simulink model "motorVelMap"  (R2016b)
settings: Solver=ode5  StartTime=0.0  StopTime=inf  FixedStep=0.001  RelTol=1e-3  EnableMultiTasking=on
undefined symbols (not defined in the file or in its folder): Humusoft, MF644
libraries: dcpctrl x2, sldrtlib x1, simulink x1
settings Model: SimulationMode=external  ExtModeArchiveMode=auto  ExtModeArchiveFileName=dsaData  ExtModeArchiveDirName=/Users/julianleland/Documents/Git/GitHub/dcpctrl_v2/data/dsaData  ExtModeIncDirWhenArm=on  Creator=julianleland  LastModifiedBy=julianleland
settings DataIOCC: SaveOutput=off  SignalLogging=off  DSMLogging=off  SaveTime=off
settings OptimizationCC: LifeSpan=inf
settings DebuggingCC: SFUnexpectedBacktrackingDiag=warning  SFNoUnconditionalDefaultTransitionDiag=warning  SFExecutionAtInitializationDiag=none
settings HardwareCC: ProdBitPerLong=64  ProdHWDeviceType=Intel->x86-64 (Mac OS X)  TargetBitPerLong=64  TargetBitPerPointer=64  TargetIntDivRoundTo=Zero  TargetEndianess=LittleEndian  TargetWordSize=64  TargetHWDeviceType=Intel->x86-64
settings RTWCC: SystemTargetFile=sldrt.tlc  TemplateMakefile=sldrt.tmf  Description=Simulink Desktop Real-Time  RTWCompilerOptimization=on
settings CodeAppCC: MaxIdLength=95
settings SimulinkDesktopRealTimeCC: TargetPreCompLibLocation=/Applications/MATLAB_R2016b.app/toolbox/sldrt/lib/maci64  TargetLangStandard=C89/C90 (ANSI)  SupportVariableSizeSignals=off
settings ConfigComp: CovMetricSettings=dw  CovHtmlReporting=on  CovSaveCumulativeToWorkspaceVar=on  CovSaveSingleToWorkspaceVar=on  CovExternalEMLEnable=off

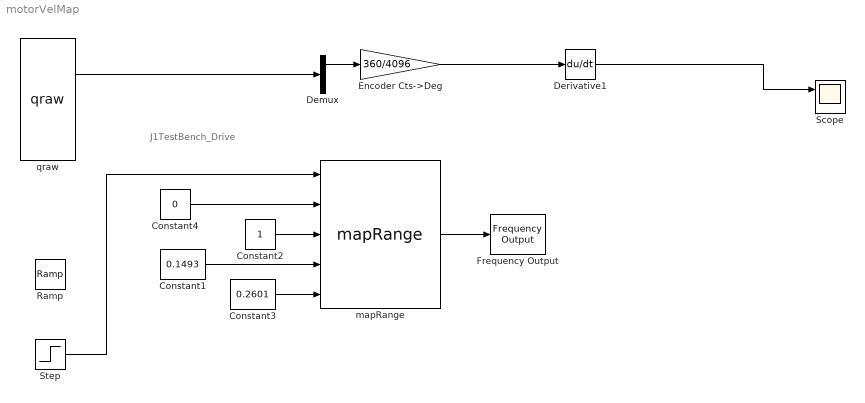
== system motorVelMap ==
  note: J1TestBench_Drive
  Constant1 : Constant  Value=0.1493
  Constant2 : Constant
  Constant3 : Constant  Value=0.2601
  Constant4 : Constant  Value=0
  Demux : Demux  Outputs=2
  Derivative1 : Derivative
  Encoder Cts->Deg : Gain  Gain=360/4096
  Frequency Output : sldrtlib/Frequency Output  SampleTime=-1  MaxMissedTicks=10  ShowMissedTicks=off  YieldWhenWaiting=off  DrvName=Humusoft/MF644  DrvAddress=4294967295  DrvOptions=585  Channels=1  FrequencySource=1  Frequency=150  FrequencyFinalValue=[]  DutySource=2  Duty=0.5  DutyFinalValue=0.5
      settings: AttributesFormatString=Humusoft\nMF644 [auto]
  Ramp : simulink/Sources/Ramp  slope=.01  start=0  X0=0
  Scope : Scope  NumInputPorts=2
  Step : Step  Time=2  Before=-1  SampleTime=0
  "mapRange " : dcpctrl/mapRange 
  qraw : dcpctrl/qraw
  wires:
  Encoder Cts->Deg/1 -> Derivative1/1
  qraw/2 -> Demux/1
  Demux/1 -> Encoder Cts->Deg/1
  Derivative1/1 -> Scope/1
  Constant2/1 -> "mapRange "/3
  Constant3/1 -> "mapRange "/5
  Constant4/1 -> "mapRange "/2
  "mapRange "/1 -> Frequency Output/1
  Constant1/1 -> "mapRange "/4
  Step/1 -> "mapRange "/1
